simulink model "LKA"  (Simulink 7.9)
settings: Solver=ode23  StartTime=0.0  StopTime=tend  FixedStep=0.01  RelTol=1e-3
undefined symbols (not defined in the file or in its folder): pin
libraries: library x6, simulink x4
settings Model: Creator=Georg  LastModifiedBy=georgnestlinger
settings OptimizationCC: InlineParams=on
settings DebuggingCC: SolverPrmCheckMsg=none  FcnCallInpInsideContextMsg=Use local settings
settings GRTTargetCC: CombineOutputUpdateFcns=off  GRTInterface=on

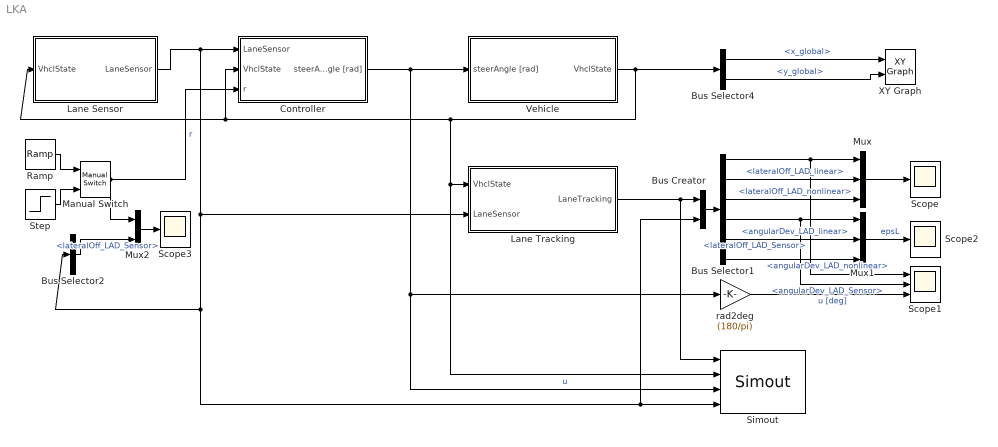
== system LKA ==
  Bus Creator : BusCreator  Inputs=2
  Bus Selector1 : BusSelector  OutputSignals=LaneSensor.lateralOff_LAD_Sensor,LaneTracking.lateralOff_LAD_linear,LaneTracking.lateralOff_LAD_nonlinear,LaneSensor.angularDev_LAD_Sensor,LaneTracking.angularDev_LAD_linear,LaneTracking.angularDev_LAD_nonlinear
  Bus Selector2 : BusSelector  OutputSignals=lateralOff_LAD_Sensor
  Bus Selector4 : BusSelector  OutputSignals=x_global,y_global
  Controller : Subsystem
  Lane Sensor : Subsystem
  Lane Tracking : Subsystem
  Manual Switch : simulink/Signal Routing/Manual Switch  sw=0  action=0  varsize=off
  Mux : Mux  Inputs=3
  Mux1 : Mux  Inputs=3
  Mux2 : Mux  Inputs=2
  Ramp : simulink/Sources/Ramp  slope=1  start=8  X0=0
  Scope : Scope
      settings: ShowLegends=on  YMin=-0.25  YMax=0.025  SaveName=ScopeData3
  Scope1 : Scope  NumInputPorts=3
      settings: TimeRange=13.0347  YMin=0~0~0  YMax=0.01~0.05~1
  Scope2 : Scope
      settings: TimeRange=13.0347  YMin=0.00932  YMax=0.009395
  Scope3 : Scope
      settings: TimeRange=5.66  YMin=0.999982  YMax=1  SaveName=ScopeData2
  Simout : library/Misc/Simout
  Step : Step  Time=10  SampleTime=0
  Vehicle : Subsystem
  XY Graph : simulink/Sinks/XY Graph  xmin=-50  xmax=700  ymin=-10  ymax=600  st=-1
  "rad2deg " : Gain  Gain=(180/pi)
  wires:
  Bus Selector4/1 -> XY Graph/1  "<x_global>"
  Bus Selector4/2 -> XY Graph/2  "<y_global>"
  Controller/1(steerAngle [rad]) -> Vehicle/1(steerAngle [rad]), Simout/3, "rad2deg "/1  "u"
  Step/1 -> Manual Switch/2
  Manual Switch/1 -> Mux2/1, Controller/3(r)  "r"
  Vehicle/1(VhclState) -> Bus Selector4/1, Controller/2(VhclState), Lane Sensor/1(VhclState), Lane Tracking/1(VhclState), Simout/2
  Mux2/1 -> Scope3/1
  Ramp/1 -> Manual Switch/1
  Lane Sensor/1(LaneSensor) -> Controller/1(LaneSensor), Lane Tracking/2(LaneSensor), Simout/4, Bus Creator/2, Bus Selector2/1
  "rad2deg "/1 -> Scope1/3  "u [deg]"
  Mux1/1 -> Scope2/1  "epsL"
  Mux/1 -> Scope/1
  Bus Selector1/1 -> Mux/1, Scope1/1  "<lateralOff_LAD_Sensor>"
  Bus Selector1/2 -> Mux/2  "<lateralOff_LAD_linear>"
  Bus Selector1/3 -> Mux/3  "<lateralOff_LAD_nonlinear>"
  Bus Selector1/4 -> Mux1/1, Scope1/2  "<angularDev_LAD_Sensor>"
  Bus Selector1/5 -> Mux1/2  "<angularDev_LAD_linear>"
  Bus Selector1/6 -> Mux1/3  "<angularDev_LAD_nonlinear>"
  Bus Creator/1 -> Bus Selector1/1
  Lane Tracking/1(LaneTracking) -> Bus Creator/1, Simout/1
  Bus Selector2/1 -> Mux2/2  "<lateralOff_LAD_Sensor>"

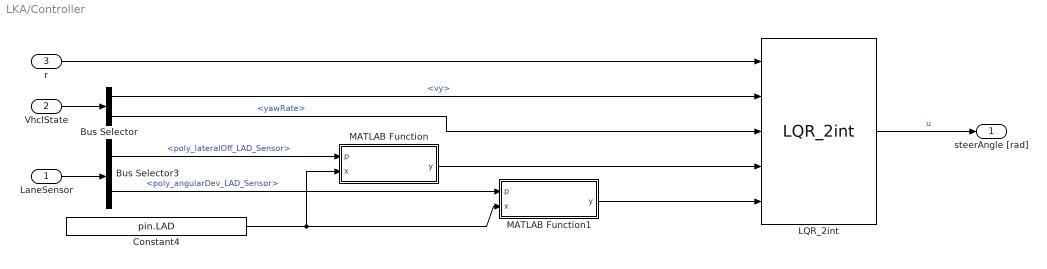
== system LKA/Controller ==
  LaneSensor : Inport
  VhclState : Inport  Port=2
  r : Inport  Port=3
  Bus Selector : BusSelector  OutputSignals=vy,yawRate
  Bus Selector3 : BusSelector  OutputSignals=poly_lateralOff_LAD_Sensor,poly_angularDev_LAD_Sensor
  Constant4 : Constant  Value=pin.LAD
  LQR_2int : library/LKA-Controller/LQR_2int
  MATLAB Function : MATLAB Function  TreatAsAtomicUnit=on
  MATLAB Function1 : MATLAB Function  TreatAsAtomicUnit=on
  steerAngle [rad] : Outport
  wires:
  r/1 -> LQR_2int/1
  MATLAB Function/1(y) -> LQR_2int/4
  MATLAB Function1/1(y) -> LQR_2int/5
  Constant4/1 -> MATLAB Function1/2(x), MATLAB Function/2(x)
  LaneSensor/1 -> Bus Selector3/1
  LQR_2int/1 -> steerAngle [rad]/1  "u"
  Bus Selector3/1 -> MATLAB Function/1(p)  "<poly_lateralOff_LAD_Sensor>"
  Bus Selector3/2 -> MATLAB Function1/1(p)  "<poly_angularDev_LAD_Sensor>"
  VhclState/1 -> Bus Selector/1
  Bus Selector/1 -> LQR_2int/2  "<vy>"
  Bus Selector/2 -> LQR_2int/3  "<yawRate>"

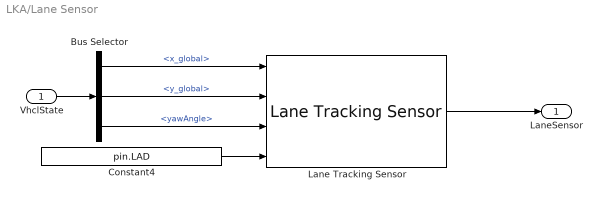
== system LKA/Lane Sensor ==
  VhclState : Inport
  Bus Selector : BusSelector  OutputSignals=x_global,y_global,yawAngle
  Constant4 : Constant  Value=pin.LAD
  Lane Tracking Sensor : library/Lane Tracking/Lane Tracking Sensor
  LaneSensor : Outport
  wires:
  Lane Tracking Sensor/1 -> LaneSensor/1
  VhclState/1 -> Bus Selector/1
  Bus Selector/1 -> Lane Tracking Sensor/1  "<x_global>"
  Bus Selector/2 -> Lane Tracking Sensor/2  "<y_global>"
  Bus Selector/3 -> Lane Tracking Sensor/3  "<yawAngle>"
  Constant4/1 -> Lane Tracking Sensor/4

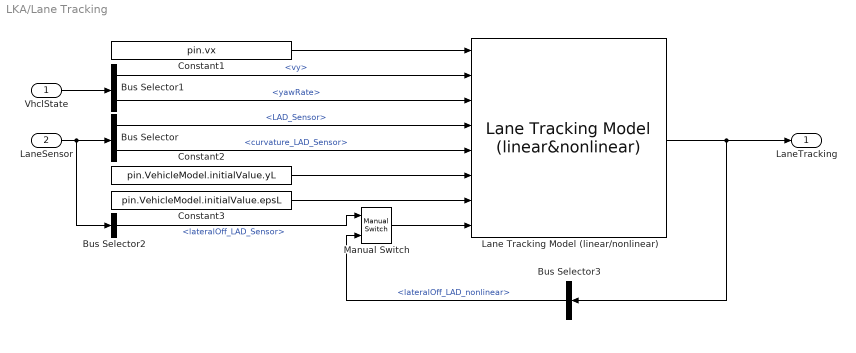
== system LKA/Lane Tracking ==
  VhclState : Inport
  LaneSensor : Inport  Port=2
  Bus Selector : BusSelector  OutputSignals=LAD_Sensor,curvature_LAD_Sensor
  Bus Selector1 : BusSelector  OutputSignals=vy,yawRate
  Bus Selector2 : BusSelector  OutputSignals=lateralOff_LAD_Sensor
  Bus Selector3 : BusSelector  OutputSignals=lateralOff_LAD_nonlinear
  Constant1 : Constant  Value=pin.vx
  Constant2 : Constant  Value=pin.VehicleModel.initialValue.yL
  Constant3 : Constant  Value=pin.VehicleModel.initialValue.epsL
  Lane Tracking Model (linear/nonlinear) : library/Lane Tracking/Lane Tracking Model (linear&nonlinear)
  Manual Switch : simulink/Signal Routing/Manual Switch  sw=1  action=0  varsize=off
  LaneTracking : Outport
  wires:
  LaneSensor/1 -> Bus Selector/1, Bus Selector2/1
  Constant2/1 -> Lane Tracking Model (linear/nonlinear)/6
  Constant3/1 -> Lane Tracking Model (linear/nonlinear)/7
  VhclState/1 -> Bus Selector1/1
  Constant1/1 -> Lane Tracking Model (linear/nonlinear)/1
  Bus Selector1/1 -> Lane Tracking Model (linear/nonlinear)/2  "<vy>"
  Bus Selector1/2 -> Lane Tracking Model (linear/nonlinear)/3  "<yawRate>"
  Bus Selector/1 -> Lane Tracking Model (linear/nonlinear)/4  "<LAD_Sensor>"
  Bus Selector/2 -> Lane Tracking Model (linear/nonlinear)/5  "<curvature_LAD_Sensor>"
  Bus Selector3/1 -> Manual Switch/2  "<lateralOff_LAD_nonlinear>"
  Bus Selector2/1 -> Manual Switch/1  "<lateralOff_LAD_Sensor>"
  Manual Switch/1 -> Lane Tracking Model (linear/nonlinear)/8
  Lane Tracking Model (linear/nonlinear)/1 -> Bus Selector3/1, LaneTracking/1

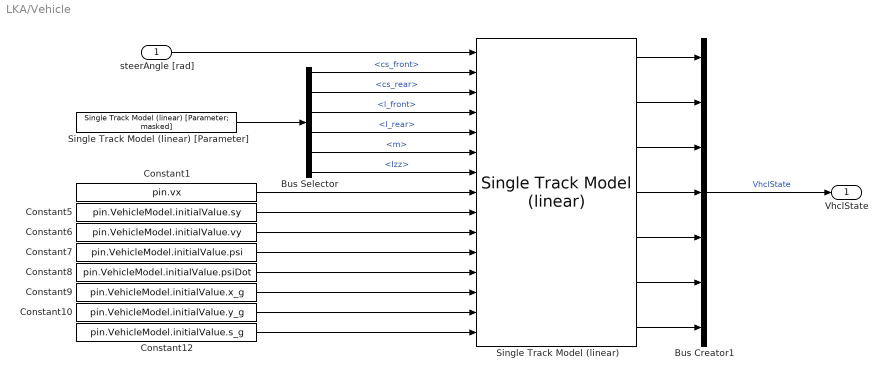
== system LKA/Vehicle ==
  steerAngle [rad] : Inport
  Bus Creator1 : BusCreator  Inputs=7
  Bus Selector : BusSelector  OutputSignals=cs_front,cs_rear,l_front,l_rear,m,Izz
  Constant1 : Constant  Value=pin.vx
  Constant10 : Constant  Value=pin.VehicleModel.initialValue.y_g
  Constant12 : Constant  Value=pin.VehicleModel.initialValue.s_g
  Constant5 : Constant  Value=pin.VehicleModel.initialValue.sy
  Constant6 : Constant  Value=pin.VehicleModel.initialValue.vy
  Constant7 : Constant  Value=pin.VehicleModel.initialValue.psi
  Constant8 : Constant  Value=pin.VehicleModel.initialValue.psiDot
  Constant9 : Constant  Value=pin.VehicleModel.initialValue.x_g
  Single Track Model (linear) : library/Vehicle Models/Single Track Models/Single Track Model (linear)
  Single Track Model (linear) [Parameter] : library/Vehicle Models ext./Single Track Model (linear) [Parameter; masked]  cs_front=pin.VehicleModel.parameter.csv  cs_rear=pin.VehicleModel.parameter.csh  l_front=pin.VehicleModel.parameter.lv  l_rear=pin.VehicleModel.parameter.lh  m=pin.VehicleModel.parameter.m  Izz=pin.VehicleModel.parameter.Iz
  VhclState : Outport
  wires:
  Constant1/1 -> Single Track Model (linear)/8
  steerAngle [rad]/1 -> Single Track Model (linear)/1
  Single Track Model (linear) [Parameter]/1 -> Bus Selector/1
  Constant5/1 -> Single Track Model (linear)/9
  Constant6/1 -> Single Track Model (linear)/10
  Constant7/1 -> Single Track Model (linear)/11
  Constant8/1 -> Single Track Model (linear)/12
  Constant9/1 -> Single Track Model (linear)/13
  Constant10/1 -> Single Track Model (linear)/14
  Constant12/1 -> Single Track Model (linear)/15
  Bus Creator1/1 -> VhclState/1  "VhclState"
  Single Track Model (linear)/1 -> Bus Creator1/1
  Single Track Model (linear)/2 -> Bus Creator1/2
  Single Track Model (linear)/3 -> Bus Creator1/3
  Single Track Model (linear)/4 -> Bus Creator1/4
  Single Track Model (linear)/5 -> Bus Creator1/5
  Single Track Model (linear)/6 -> Bus Creator1/6
  Single Track Model (linear)/7 -> Bus Creator1/7
  Bus Selector/1 -> Single Track Model (linear)/2  "<cs_front>"
  Bus Selector/2 -> Single Track Model (linear)/3  "<cs_rear>"
  Bus Selector/3 -> Single Track Model (linear)/4  "<l_front>"
  Bus Selector/4 -> Single Track Model (linear)/5  "<l_rear>"
  Bus Selector/5 -> Single Track Model (linear)/6  "<m>"
  Bus Selector/6 -> Single Track Model (linear)/7  "<Izz>"

== matlab function Controller/MATLAB Function ==
  data: p input double; y output double; x input double
function y = polyVal(p,x)
%#codegen

y = polyval(p,x);

== matlab function Controller/MATLAB Function1 ==
  data: p input double; y output double; x input double
function y = polyVal(p,x)
%#codegen

y = polyval(p,x);
